simulink model "testBufferModelErrorCompensator"  (R2015a)
settings: Solver=ode4  StartTime=0.0  StopTime=20  FixedStep=0.016  RelTol=1e-3
libraries: simulink x1
settings Model: Creator=go  LastModifiedBy=go

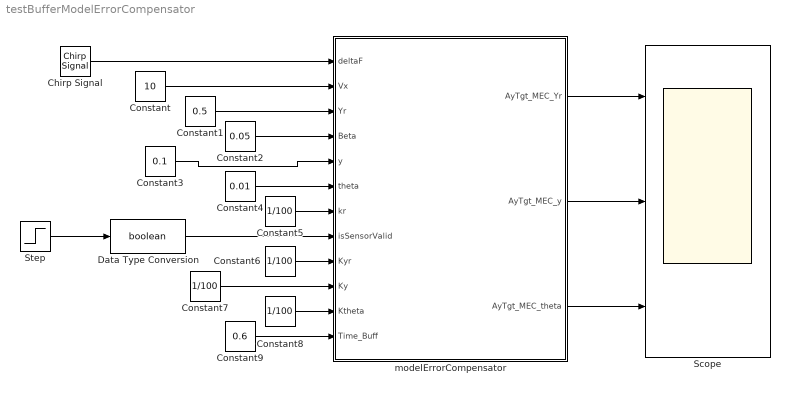
== system testBufferModelErrorCompensator ==
  Chirp Signal : simulink/Sources/Chirp Signal  f1=0.1  T=100  f2=1
  Constant : Constant  Value=10
  Constant1 : Constant  Value=0.5
  Constant2 : Constant  Value=0.05
  Constant3 : Constant  Value=0.1
  Constant4 : Constant  Value=0.01
  Constant{5..8} (4 alike) : Constant  Value=1/100
  Constant9 : Constant  Value=0.6
  Data Type Conversion : DataTypeConversion  OutDataTypeStr=boolean
  Scope : Scope  NumInputPorts=3
      settings: YMin=-5~-5~-5  YMax=5~5~5
  Step : Step  Time=0.5  SampleTime=0
  modelErrorCompensator : MATLAB Function  TreatAsAtomicUnit=on
  wires:
  Chirp Signal/1 -> modelErrorCompensator/1(deltaF)
  Data Type Conversion/1 -> modelErrorCompensator/8(isSensorValid)
  modelErrorCompensator/1(AyTgt_MEC_Yr) -> Scope/1
  modelErrorCompensator/2(AyTgt_MEC_y) -> Scope/2
  Step/1 -> Data Type Conversion/1
  modelErrorCompensator/3(AyTgt_MEC_theta) -> Scope/3
  Constant/1 -> modelErrorCompensator/2(Vx)
  Constant1/1 -> modelErrorCompensator/3(Yr)
  Constant2/1 -> modelErrorCompensator/4(Beta)
  Constant3/1 -> modelErrorCompensator/5(y)
  Constant4/1 -> modelErrorCompensator/6(theta)
  Constant5/1 -> modelErrorCompensator/7(kr)
  Constant6/1 -> modelErrorCompensator/9(Kyr)
  Constant7/1 -> modelErrorCompensator/10(Ky)
  Constant8/1 -> modelErrorCompensator/11(Ktheta)
  Constant9/1 -> modelErrorCompensator/12(Time_Buff)

== matlab function testBufferModelErrorCompensator/modelErrorCompensator ==
  data: deltaF input; Vx input; AyTgt_MEC_Yr output; AyTgt_MEC_y output; Yr input; Beta input; y input; theta input; kr input; isSensorValid input; Kyr input; Ky input; Ktheta input; Time_Buff input; AyTgt_MEC_theta output
function [ AyTgt_MEC_Yr,AyTgt_MEC_y, AyTgt_MEC_theta] = modelErrorCompensator( deltaF,Vx, Yr , Beta , y ,theta , kr, isSensorValid ,Kyr,Ky,Ktheta,Time_Buff)
% MODELERRORCOMPENSATOR Summary of this function goes here
% Detailed explanation goes here

% ToDo  
% Modifiy theta dyamics 

[ Yr_est, Beta_est, y_est, theta_est,isEstCompleated ] = imposedDynamicsEstimator( deltaF, Vx , Yr , Beta , y ,theta , kr, isSensorValid,Time_Buff);

if isEstCompleated == true
  AyTgt_MEC_Yr    =   Kyr    * ( Yr_est       - Yr    );
  AyTgt_MEC_y     = - Ky     * ( y_est        - y     );
  AyTgt_MEC_theta = - Ktheta * ( theta_est    - theta );
else
  AyTgt_MEC_Yr    = 0;
  AyTgt_MEC_y     = 0;
  AyTgt_MEC_theta = 0;
end

end
